simulink library "CHP_Model_lib"  (Simulink 8.1)
settings: Solver=ode45  StartTime=0.0  StopTime=10.0  RelTol=1e-3
undefined symbols (not defined in the file): DiscIntNeverNeededParam, SIM_HIL, Ts
libraries: simulink x1, dsparch4 x1
settings Model: Creator=re25624  LastModifiedBy=re25624

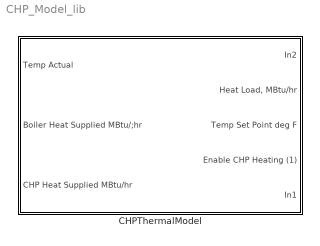
== system CHP_Model_lib ==
  CHPThermalModel : Subsystem  mask{SIM_HIL=SIM_HIL}
      mask prompts: SIM_HIL "SIM_HIL [Selects Opal-RT(1) or Simulink(0)]"

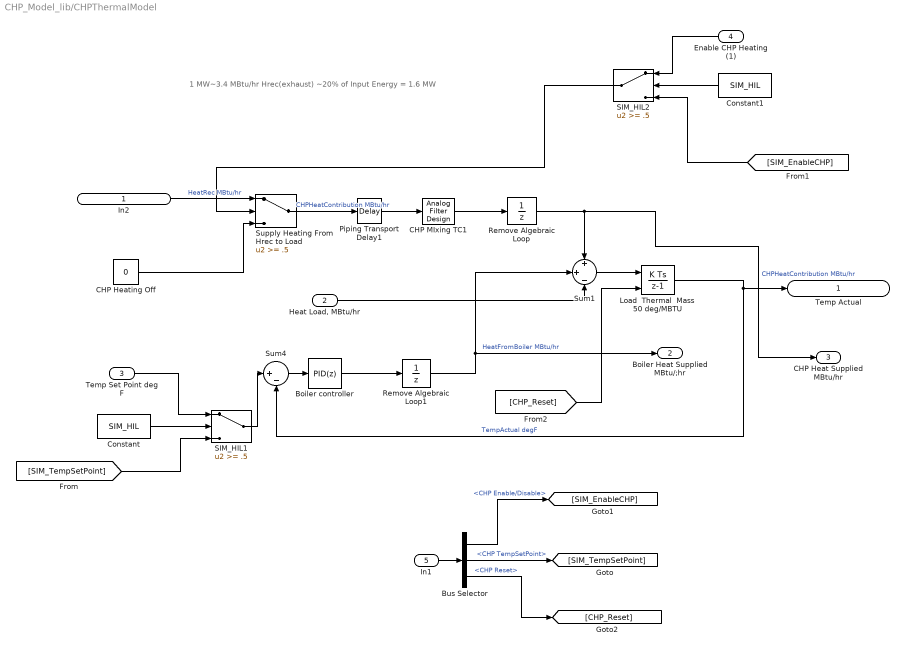
== system CHP_Model_lib/CHPThermalModel ==
  note: 1 MW~3.4 MBtu/hr
      | Hrec(exhaust) ~20% of Input Energy = 1.6 MW
  In2 : Inport
  "Heat Load, MBtu/hr" : Inport  Port=2
  Temp Set Point deg F : Inport  Port=3
  Enable CHP Heating (1) : Inport  Port=4
  In1 : Inport  Port=5
  Boiler controller : simulink/Continuous/PID Controller  Controller=PID  TimeDomain=Discrete-time  SampleTime=-1  IntegratorMethod=Forward Euler  FilterMethod=Forward Euler  Form=Parallel  P=100  I=.01  D=0  N=100  InitialConditionSource=internal  InitialConditionForIntegrator=0  InitialConditionForFilter=0  ExternalReset=none  LimitOutput=on  UpperSaturationLimit=20  LowerSaturationLimit=0  LinearizeAsGain=on  AntiWindupMode=none  Kb=1  TrackingMode=off  Kt=1  PParamMin=[]  PParamMax=[]  IParamMin=[]  IParamMax=[]  DParamMin=[]  DParamMax=[]  NParamMin=[]  NParamMax=[]  KbParamMin=[]  KbParamMax=[]  KtParamMin=[]  KtParamMax=[]  POutMin=[]  POutMax=[]  IOutMin=[]  IOutMax=[]  DOutMin=[]  DOutMax=[]  NOutMin=[]  NOutMax=[]  KbOutMin=[]  KbOutMax=[]  KtOutMin=[]  KtOutMax=[]  IntegratorOutMin=[]  IntegratorOutMax=[]  FilterOutMin=[]  FilterOutMax=[]  SumOutMin=[]  SumOutMax=[]  SumI1OutMin=[]  SumI1OutMax=[]  SumI2OutMin=[]  SumI2OutMax=[]  SumI3OutMin=[]  SumI3OutMax=[]  SumDOutMin=[]  SumDOutMax=[]  SaturationOutMin=[]  SaturationOutMax=[]  IntegratorContinuousStateAttributes=''  IntegratorStateMustResolveToSignalObject=off  IntegratorRTWStateStorageClass=Auto  FilterContinuousStateAttributes=''  FilterStateMustResolveToSignalObject=off  FilterRTWStateStorageClass=Auto
  Bus Selector : BusSelector  OutputSignals=CHP Enable/Disable,CHP TempSetPoint,CHP Reset
  CHP Heating Off : Constant  Value=0  SampleTime=Ts
  CHP MIxing TC1 : dsparch4/Analog Filter Design  method=Butterworth  filttype=Lowpass  N=2  Wlo=0.2*pi  Whi=80  Rp=2  Rs=40
  Constant : Constant  Value=SIM_HIL
  Constant1 : Constant  Value=SIM_HIL
  Load  Thermal  Mass 50 deg/MBTU : DiscreteIntegrator  gainval=50/3600  ExternalReset=level  InitialCondition=20  SampleTime=-1  ICPrevOutput=DiscIntNeverNeededParam  ICPrevScaledInput=DiscIntNeverNeededParam
  Piping Transport Delay1 : TransportDelay  DelayTime=10
  Remove Algebraic Loop : UnitDelay  SampleTime=-1
  Remove Algebraic Loop1 : UnitDelay  SampleTime=-1
  SIM_HIL1 : Switch  Threshold=.5
  SIM_HIL2 : Switch  Threshold=.5
  Sum1 : Sum  Inputs=+|+|-
  Sum4 : Sum  Inputs=|+-
  Supply Heating From Hrec to Load : Switch  Threshold=.5
  Temp Actual : Outport
  Boiler Heat Supplied MBtu/;hr : Outport  Port=2
  CHP Heat Supplied MBtu/hr : Outport  Port=3
  wires:
  CHP MIxing TC1/1 -> Remove Algebraic Loop/1
  Piping Transport Delay1/1 -> CHP MIxing TC1/1
  CHP Heating Off/1 -> Supply Heating From Hrec to Load/3
  Bus Selector/2 -> [SIM_TempSetPoint]  "<CHP TempSetPoint>"
  Bus Selector/3 -> [CHP_Reset]  "<CHP Reset>"
  Bus Selector/1 -> [SIM_EnableCHP]  "<CHP Enable/Disable>"
  In1/1 -> Bus Selector/1
  Constant1/1 -> SIM_HIL2/2
  Constant/1 -> SIM_HIL1/2
  SIM_HIL2/1 -> Supply Heating From Hrec to Load/2
  [SIM_EnableCHP] -> SIM_HIL2/3
  SIM_HIL1/1 -> Sum4/1
  [SIM_TempSetPoint] -> SIM_HIL1/3
  Temp Set Point deg F/1 -> SIM_HIL1/1
  Remove Algebraic Loop/1 -> Sum1/1, CHP Heat Supplied MBtu/hr/1  "CHPHeatContribution MBtu/hr"
  Remove Algebraic Loop1/1 -> Sum1/2, Boiler Heat Supplied MBtu/;hr/1  "HeatFromBoiler MBtu/hr"
  Supply Heating From Hrec to Load/1 -> Piping Transport Delay1/1  "CHPHeatContribution MBtu/hr"
  Enable CHP Heating (1)/1 -> SIM_HIL2/1
  In2/1 -> Supply Heating From Hrec to Load/1  "HeatRec MBtu/hr"
  [CHP_Reset] -> Load  Thermal  Mass 50 deg/MBTU/2
  Load  Thermal  Mass 50 deg/MBTU/1 -> Temp Actual/1, Sum4/2  "TempActual degF"
  Sum1/1 -> Load  Thermal  Mass 50 deg/MBTU/1
  Boiler controller/1 -> Remove Algebraic Loop1/1
  Sum4/1 -> Boiler controller/1
  "Heat Load, MBtu/hr"/1 -> Sum1/3
